simulink model "ejh62a"  (Simulink 3.00)
settings: Solver=ode45  StartTime=0.0  StopTime=10.0  RelTol=1e-3
values from neighbouring files (symbols this model uses):
  s = u( (5*n+1):(6*n) )    [adapli.m]
  x = P_global(1,:)'    [contp5.m]    (also in ejh31.m = [0:0.2:5]; ejh62.m = 0:0.01:12; ejh63.m = 0:0.01:12)
  y = P_global(2,:)'    [contp5.m]    (also in ejh31.m = sqrt(25-x.^2); ejh62.m = 0:0.01:12; ejh63.m = 0:0.01:12)
libraries: HEMERO x2
settings Model: LastModifiedBy=Administrador

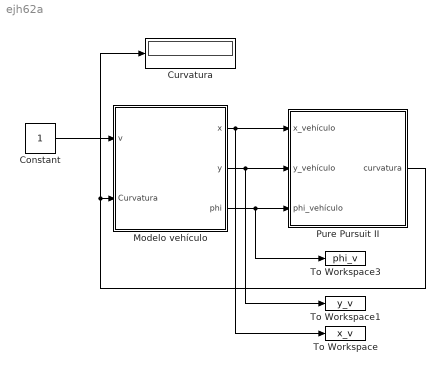
== system ejh62a ==
  Constant : Constant  Value=1
  Curvatura : Display
      settings: Format=short
  Modelo vehículo : Subsystem  mask{x_inicial=0, y_inicial=0.5, phi_inicial=0}
      mask prompts: x_inicial "Valor inicial de la coordenada x:"; y_inicial "Valor inicial de la coordenada y:"; phi_inicial "Valor inicial de la orientación:"
  Pure Pursuit II : Subsystem  mask(Pure Pursuit II){x_camino=x, y_camino=y, s=s}
      mask prompts: x_camino "Coordenadas x del camino:"; y_camino "Coordenadas y del camino:"; s "Distancia sobre el camino (s):"
      mask help: Este bloque se encarga de calcular la curvatura que es necesario suministrar al vehículo cuando se emplea la técnica de persecución pura con el parámetro look-ahead (L) variable en función del punto objetivo.
      mask init:
      | global K_ANT
      | global INDEX
      | K_ANT=1;
      | for k=1:length(x_camino)-1
      |    acum(k)=0;
      |    for w=k:length(x_camino)-1
      |       dist_entre_puntos=sqrt( (x_camino(w)-x_camino(w+1))^2 + (y_camino(w)-y_camino(w+1))^2 );
      |       acum(w+1)=acum(w)+dist_entre_puntos;
      |    end
      |    dif=abs(acum-s);
      |    [z,indice] = min(dif);
      |    INDEX(k)=indice;
      | end
  To Workspace : ToWorkspace  VariableName=x_v  SampleTime=-1  SaveFormat=Matrix
  To Workspace1 : ToWorkspace  VariableName=y_v  SampleTime=-1  SaveFormat=Matrix
  To Workspace3 : ToWorkspace  VariableName=phi_v  SampleTime=-1  SaveFormat=Matrix
  wires:
  Constant/1 -> Modelo vehículo/1(v)
  Modelo vehículo/1(x) -> To Workspace/1, Pure Pursuit II/1(x_vehículo)
  Pure Pursuit II/1(curvatura) -> Modelo vehículo/2(Curvatura), Curvatura/1
  Modelo vehículo/2(y) -> To Workspace1/1, Pure Pursuit II/2(y_vehículo)
  Modelo vehículo/3(phi) -> Pure Pursuit II/3(phi_vehículo), To Workspace3/1

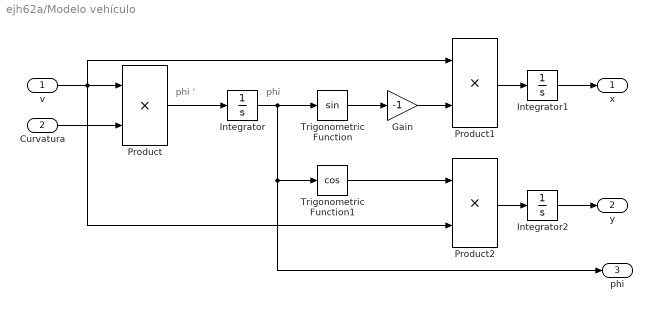
== system ejh62a/Modelo vehículo ==
  note: phi '
  note: phi
  v : Inport  Port=1  PortWidth=-1  SampleTime=-1  DataType=auto
      settings: SignalType=auto
  Curvatura : Inport  Port=2  PortWidth=-1  SampleTime=-1  DataType=auto
      settings: SignalType=auto
  Gain : Gain  Gain=-1  SaturateOnIntegerOverflow=on
  Integrator : Integrator  ExternalReset=none  InitialConditionSource=internal  InitialCondition=phi_inicial  LimitOutput=off  UpperSaturationLimit=inf  LowerSaturationLimit=-inf  ShowSaturationPort=off  ShowStatePort=off  AbsoluteTolerance=auto
  Integrator1 : Integrator  ExternalReset=none  InitialConditionSource=internal  InitialCondition=x_inicial  LimitOutput=off  UpperSaturationLimit=inf  LowerSaturationLimit=-inf  ShowSaturationPort=off  ShowStatePort=off  AbsoluteTolerance=auto
  Integrator2 : Integrator  ExternalReset=none  InitialConditionSource=internal  InitialCondition=y_inicial  LimitOutput=off  UpperSaturationLimit=inf  LowerSaturationLimit=-inf  ShowSaturationPort=off  ShowStatePort=off  AbsoluteTolerance=auto
  Product : Product  Inputs=2  SaturateOnIntegerOverflow=on
  Product1 : Product  Inputs=2  SaturateOnIntegerOverflow=on
  Product2 : Product  Inputs=2  SaturateOnIntegerOverflow=on
  Trigonometric Function : Trigonometry  Operator=sin  OutputSignalType=auto
  Trigonometric Function1 : Trigonometry  Operator=cos  OutputSignalType=auto
  x : Outport  Port=1
  y : Outport  Port=2
  phi : Outport  Port=3
  wires:
  Curvatura/1 -> Product/2
  Product/1 -> Integrator/1
  Integrator/1 -> Trigonometric Function/1, Trigonometric Function1/1, phi/1
  Trigonometric Function/1 -> Gain/1
  Gain/1 -> Product1/2
  v/1 -> Product/1, Product1/1, Product2/2
  Trigonometric Function1/1 -> Product2/1
  Product1/1 -> Integrator1/1
  Product2/1 -> Integrator2/1
  Integrator2/1 -> y/1
  Integrator1/1 -> x/1

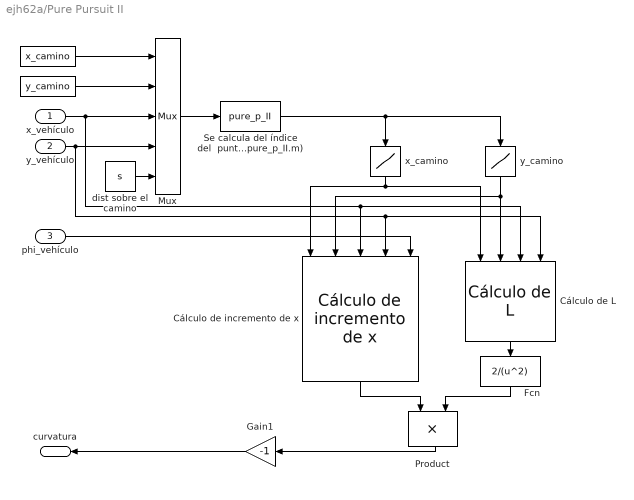
== system ejh62a/Pure Pursuit II ==
  x_vehículo : Inport  Port=1  PortWidth=-1  SampleTime=-1  DataType=auto
      settings: SignalType=auto
  y_vehículo : Inport  Port=2  PortWidth=-1  SampleTime=-1  DataType=auto
      settings: SignalType=auto
  phi_vehículo : Inport  Port=3  PortWidth=-1  SampleTime=-1  DataType=auto
      settings: SignalType=auto
  " " : Constant  Value=y_camino
  "  " : Constant  Value=x_camino
  Cálculo de L : HEMERO/Robots móviles/Control de robots móviles/Métodos geométricos/Pure Pursuit II/Cálculo de L  Orientation=down
  Cálculo de incremento de x : HEMERO/Robots móviles/Control de robots móviles/Métodos geométricos/Pure Pursuit II/Cálculo de incremento de x  Orientation=down
  Fcn : Fcn  Orientation=down  Expr=2/(u^2)
  Gain1 : Gain  Orientation=left  Gain=-1  SaturateOnIntegerOverflow=on
  Mux : Mux  Inputs=5
      settings: DisplayOption=none
  Product : Product  Orientation=down  Inputs=2  SaturateOnIntegerOverflow=on
  Se calcula del índice del  punto que está a distancia s sobre el camino desde el  punto del camino más próximo (pure_p_II.m) : MATLABFcn  MATLABFcn=pure_p_II  OutputWidth=-1  OutputSignalType=auto
  dist sobre el camino : Constant  Value=s
  x_camino : Lookup  Orientation=down  InputValues=1:length(x_camino)  OutputValues=x_camino
  y_camino : Lookup  Orientation=down  InputValues=1:length(y_camino)  OutputValues=y_camino
  curvatura : Outport  Orientation=left  Port=1
  wires:
  Se calcula del índice del  punto que está a distancia s sobre el camino desde el  punto del camino más próximo (pure_p_II.m)/1 -> y_camino/1, x_camino/1
  Gain1/1 -> curvatura/1
  Product/1 -> Gain1/1
  "  "/1 -> Mux/1
  " "/1 -> Mux/2
  x_vehículo/1 -> Mux/3, Cálculo de incremento de x/3, Cálculo de L/3
  y_vehículo/1 -> Mux/4, Cálculo de incremento de x/4, Cálculo de L/4
  dist sobre el camino/1 -> Mux/5
  Mux/1 -> Se calcula del índice del  punto que está a distancia s sobre el camino desde el  punto del camino más próximo (pure_p_II.m)/1
  Cálculo de incremento de x/1 -> Product/1
  phi_vehículo/1 -> Cálculo de incremento de x/5
  Fcn/1 -> Product/2
  Cálculo de L/1 -> Fcn/1
  y_camino/1 -> Cálculo de incremento de x/2, Cálculo de L/2
  x_camino/1 -> Cálculo de incremento de x/1, Cálculo de L/1
